simulink subsystem "Combustion_Model"  (R2020b)
settings: Solver=VariableStepAuto  StartTime=0.0  StopTime=10.0  RelTol=1e-3
undefined symbols (not defined in the file or in its folder): sim
settings Model: Creator=Edward  LastModifiedBy=Edward

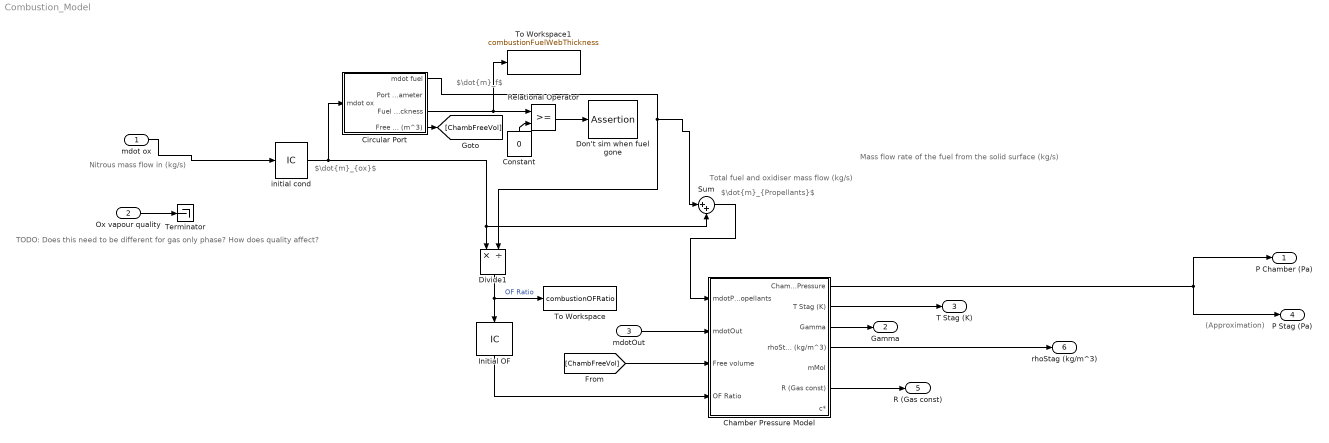
== system Combustion_Model ==
  note: (Approximation)
  note: $\dot{m}_f$
  note: $\dot{m}_{ox}$
  note: $\dot{m}_{Propellants}$
  note: TODO: Does this need to be different for gas only phase? How does quality affect?
  note: Total fuel and oxidiser mass flow (kg/s)
  note: Mass flow rate of the fuel from the solid surface (kg/s)
  note: Nitrous mass flow in (kg/s)
  mdot ox : Inport
  Ox vapour quality : Inport  Port=2
  mdotOut : Inport  Port=3
  Chamber Pressure Model : Subsystem
  Circular Port : Subsystem
  Constant : Constant  Value=0
  Divide1 : Product  Inputs=*/
  Don't sim when fuel gone : Assertion
  "Initial OF " : InitialCondition  Value=sim.combustionChamber.OFRatioInitial
  Relational Operator : RelationalOperator  OutDataTypeStr=boolean  RndMeth=Simplest
  Sum : Sum  Inputs=|++
  Terminator : Terminator
  To Workspace : ToWorkspace  VariableName=combustionOFRatio  SaveFormat=Timeseries  SampleTime=-1
  To Workspace1 : ToWorkspace  VariableName=combustionFuelWebThickness  SaveFormat=Timeseries  SampleTime=-1
  initial cond : InitialCondition  Value=sim.combustionChamber.mdotOxInitial
  P Chamber (Pa) : Outport
  Gamma : Outport  Port=2
  T Stag (K) : Outport  Port=3
  "P Stag (Pa) " : Outport  Port=4
  R (Gas const) : Outport  Port=5
  rhoStag (kg/m^3) : Outport  Port=6
  wires:
  Sum/1 -> Chamber Pressure Model/1(mdotPropellants)
  Circular Port/3(Fuel web thickness) -> Relational Operator/1, To Workspace1/1
  Constant/1 -> Relational Operator/2
  Relational Operator/1 -> Don't sim when fuel gone/1
  Circular Port/1(mdot fuel) -> Sum/1, Divide1/2
  "Initial OF "/1 -> Chamber Pressure Model/4(OF Ratio)
  initial cond/1 -> Divide1/1, Sum/2, Circular Port/1(mdot ox)
  Divide1/1 -> "Initial OF "/1, To Workspace/1  "OF Ratio"
  Ox vapour quality/1 -> Terminator/1
  Circular Port/4(Free volume (m^3)) -> [ChambFreeVol]
  mdot ox/1 -> initial cond/1
  Chamber Pressure Model/1(Chamber Pressure) -> "P Stag (Pa) "/1, P Chamber (Pa)/1
  mdotOut/1 -> Chamber Pressure Model/2(mdotOut)
  [ChambFreeVol] -> Chamber Pressure Model/3(Free volume)
  Chamber Pressure Model/2(T Stag (K)) -> T Stag (K)/1
  Chamber Pressure Model/3(Gamma) -> Gamma/1
  Chamber Pressure Model/4(rhoStag (kg/m^3)) -> rhoStag (kg/m^3)/1
  Chamber Pressure Model/6(R (Gas const)) -> R (Gas const)/1

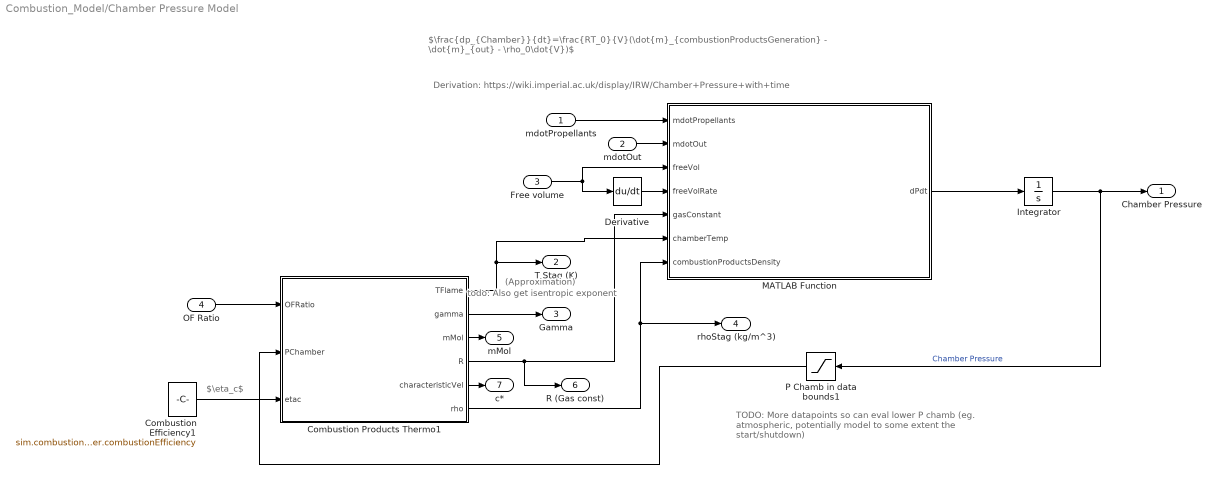
== system Combustion_Model/Chamber Pressure Model ==
  note: TODO: More datapoints
      | so can eval lower P chamb (eg. atmospheric, potentially
      | model to some extent the start/shutdown)
  note: $\eta_c$
  note: (Approximation)
  note: todo: Also get isentropic exponent
  note: $\frac{dp_{Chamber}}{dt}=\frac{RT_0}{V}(\dot{m}_{combustionProductsGeneration} - \dot{m}_{out} - \rho_0\dot{V})$
  note: Derivation: https://wiki.imperial.ac.uk/display/IRW/Chamber+Pressure+with+time
  mdotPropellants : Inport
  mdotOut : Inport  Port=2
  Free volume : Inport  Port=3
  OF Ratio : Inport  Port=4
  Combustion Efficiency1 : Constant  Value=sim.combustionChamber.combustionEfficiency
  Combustion Products Thermo1 : MATLAB Function  TreatAsAtomicUnit=on
  Derivative : Derivative
  Integrator : Integrator  InitialCondition=sim.combustionChamber.PChamberInit
  MATLAB Function : MATLAB Function  TreatAsAtomicUnit=on
  P Chamb in data bounds1 : Saturate  UpperLimit=45e5  LowerLimit=15.1e5
  Chamber Pressure : Outport
  T Stag (K) : Outport  Port=2
  Gamma : Outport  Port=3
  rhoStag (kg/m^3) : Outport  Port=4
  mMol : Outport  Port=5
  R (Gas const) : Outport  Port=6
  c* : Outport  Port=7
  wires:
  Combustion Products Thermo1/3(mMol) -> mMol/1
  mdotPropellants/1 -> MATLAB Function/1(mdotPropellants)
  Combustion Products Thermo1/5(characteristicVel) -> c*/1
  Free volume/1 -> MATLAB Function/3(freeVol), Derivative/1
  Combustion Products Thermo1/6(rho) -> MATLAB Function/7(combustionProductsDensity), rhoStag (kg/m^3)/1
  Combustion Products Thermo1/1(TFlame) -> MATLAB Function/6(chamberTemp), T Stag (K)/1
  Combustion Products Thermo1/4(R) -> MATLAB Function/5(gasConstant), R (Gas const)/1
  Combustion Efficiency1/1 -> Combustion Products Thermo1/3(etac)
  OF Ratio/1 -> Combustion Products Thermo1/1(OFRatio)
  Derivative/1 -> MATLAB Function/4(freeVolRate)
  Combustion Products Thermo1/2(gamma) -> Gamma/1
  mdotOut/1 -> MATLAB Function/2(mdotOut)
  MATLAB Function/1(dPdt) -> Integrator/1
  Integrator/1 -> P Chamb in data bounds1/1, Chamber Pressure/1  "Chamber Pressure"
  P Chamb in data bounds1/1 -> Combustion Products Thermo1/2(PChamber)

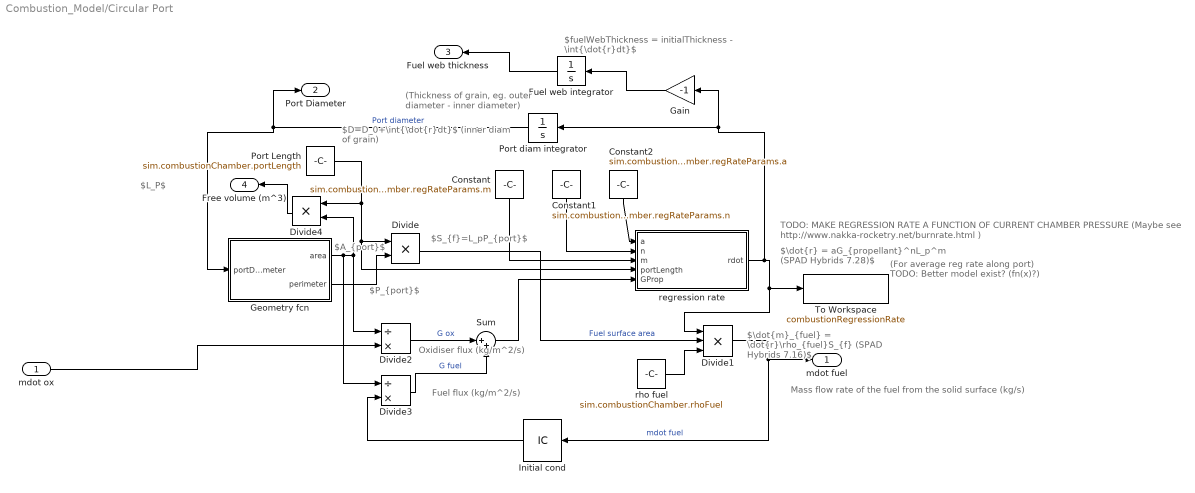
== system Combustion_Model/Circular Port ==
  note: Fuel flux (kg/m^2/s)
  note: Mass flow rate of the fuel from the solid surface (kg/s)
  note: $\dot{r} = aG_{propellant}^nL_p^m (SPAD Hybrids 7.28)$
  note: (For average reg rate along port)
      | TODO: Better model exist? (fn(x)?)
  note: $L_P$
  note: $D=D_0+\int{\dot{r}dt}$ (inner diam of grain)
  note: $fuelWebThickness = initialThickness - \int{\dot{r}dt}$
  note: (Thickness of grain, eg. outer
      | diameter - inner diameter)
  note: Oxidiser flux (kg/m^2/s)
  note: $\dot{m}_{fuel} = \dot{r}\rho_{fuel}S_{f} (SPAD Hybrids 7.16)$
  note: $P_{port}$
  note: $A_{port}$
  note: $S_{f}=L_pP_{port}$
  note: TODO: MAKE REGRESSION RATE A FUNCTION OF CURRENT CHAMBER PRESSURE (Maybe see http://www.nakka-rocketry.net/burnrate.html )
  mdot ox : Inport
  Constant : Constant  Value=sim.combustionChamber.regRateParams.m
  Constant1 : Constant  Value=sim.combustionChamber.regRateParams.n
  Constant2 : Constant  Value=sim.combustionChamber.regRateParams.a
  Divide : Product  Inputs=**
  Divide1 : Product  Inputs=***
  Divide2 : Product  Inputs=/*
  Divide3 : Product  Inputs=/*
  Divide4 : Product  Inputs=**
  "Fuel web integrator " : Integrator  InitialCondition=sim.combustionChamber.initialFuelWebThickness
  Gain : Gain  Gain=-1
  "Geometry fcn " : MATLAB Function  TreatAsAtomicUnit=on
  Initial cond : InitialCondition  Value=sim.combustionChamber.mdotOxInitial / sim.combustionChamber.OFRatioInitial
  Port Length : Constant  Value=sim.combustionChamber.portLength
  Port diam integrator : Integrator  InitialCondition=sim.combustionChamber.initialPortDiameter
  Sum : Sum  Inputs=|++
  To Workspace : ToWorkspace  VariableName=combustionRegressionRate  SaveFormat=Timeseries  SampleTime=-1
  regression rate : MATLAB Function  TreatAsAtomicUnit=on
  rho fuel : Constant  Value=sim.combustionChamber.rhoFuel
  mdot fuel : Outport
  Port Diameter : Outport  Port=2
  Fuel web thickness : Outport  Port=3
  Free volume (m^3) : Outport  Port=4
  wires:
  Divide4/1 -> Free volume (m^3)/1
  "Geometry fcn "/2(perimeter) -> Divide/2
  Initial cond/1 -> Divide3/2
  Constant2/1 -> regression rate/1(a)
  Constant1/1 -> regression rate/2(n)
  Constant/1 -> regression rate/3(m)
  "Fuel web integrator "/1 -> Fuel web thickness/1
  Gain/1 -> "Fuel web integrator "/1
  regression rate/1(rdot) -> Divide1/1, To Workspace/1, Port diam integrator/1, Gain/1
  Port diam integrator/1 -> Port Diameter/1, "Geometry fcn "/1(portDiameter)  "Port diameter"
  Sum/1 -> regression rate/5(GProp)
  mdot ox/1 -> Divide2/2
  Divide2/1 -> Sum/1  "G ox"
  Divide3/1 -> Sum/2  "G fuel"
  Divide1/1 -> Initial cond/1, mdot fuel/1  "mdot fuel"
  rho fuel/1 -> Divide1/3
  Divide/1 -> Divide1/2  "Fuel surface area"
  "Geometry fcn "/1(area) -> Divide4/2, Divide2/1, Divide3/1
  Port Length/1 -> Divide/1, regression rate/4(portLength), Divide4/1

== matlab function Combustion_Model/Circular Port/Geometry fcn  ==
  data: portDiameter input; area output; perimeter output
function [area, perimeter] = fcn(portDiameter)
area = pi.*(portDiameter./2).^2;
perimeter = pi.*portDiameter;

== matlab function Combustion_Model/Circular Port/regression rate ==
  data: a input; n input; m input; portLength input; rdot output; GProp input
function rdot = regressionRate(a, n, m, portLength, GProp)
rdot = a.*(GProp.^n).*portLength.^m;

== matlab function Combustion_Model/Chamber Pressure Model/MATLAB Function ==
  data: mdotPropellants input; dPdt output; mdotOut input; freeVol input; freeVolRate input; gasConstant input; chamberTemp input; combustionProductsDensity input
function dPdt = chamberPressureRate(mdotPropellants, mdotOut, ...
    freeVol, freeVolRate, gasConstant, chamberTemp, combustionProductsDensity)
%Unsteady combustion chamber pressure
%
%Inputs:
%mdotPropellants = Rate of combustion products generation (kg/s)
%mdotOut = Rate of combustion products leaving chamber (kg/s)
%freeVol = Instantaneous free volume in the chamber (m^3)
%freeVolRate = Time rate of change of freeVol (m^3/s)
%gasConstant = Gas specific constant (Eg. 287 for air) of combustion
%products
%chamberTemp = Temp of combustion chamber, often taken to be adiabatic
%flame temp (K)
%combustionProductsDensity = Density of combustion products (kg/m^3)
%
%Assumptions:
%-Relationship between pressure change rate and density change rate given
%by ideal gas law
%-Similar derivation to: http://www.nakka-rocketry.net/th_pres.html#Pressure
dPdt = ((gasConstant.*chamberTemp)./freeVol) .* (mdotPropellants - mdotOut - combustionProductsDensity.*freeVolRate);

== matlab function Combustion_Model/Chamber Pressure Model/Combustion Products Thermo1 ==
  data: OFRatio input; TFlame output; PChamber input; etac input; gamma output; mMol output; R output; characteristicVel output; propepProps parameter; rho output
function [TFlame, gamma, mMol, R, characteristicVel, rho] = combustionProductsProperties(OFRatio, PChamber, etac, propepProps)
%Keep within data. TODO: Expand dataset
if(OFRatio > 10)
   OFRatio = 10; 
end
if(OFRatio < 2.003)
   OFRatio = 2.003; 
end
[TFlame, gamma, mMol, R, characteristicVel] = HybridMotor.thermochem(propepProps, OFRatio, PChamber, etac);
%Assume ideal gas:
%P = rho*R*T -> rho = P/(R*T)
rho = PChamber ./ (R.*TFlame);
